simulink model "switch_basic"  (Simulink 6.6)
settings: Solver=FixedStepDiscrete  StartTime=0.0  StopTime=10.0  FixedStep=1  RelTol=1e-3
settings Model: Creator=ksmyth  LastModifiedBy=hnine

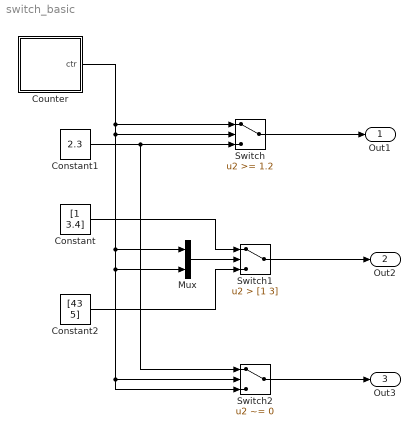
== system switch_basic ==
  Constant : Constant  Value=[1 3.4]
  Constant1 : Constant  Value=2.3
  Constant2 : Constant  Value=[43 5]
  Counter : Stateflow chart
  Mux : Mux  Inputs=2
  Switch : Switch  Threshold=1.2
  Switch1 : Switch  Criteria=u2 > Threshold  Threshold=[1 3]
  Switch2 : Switch  Criteria=u2 ~= 0
  Out1 : Outport
  Out2 : Outport  Port=2
  Out3 : Outport  Port=3
  wires:
  Constant1/1 -> Switch/3, Switch2/1
  Constant/1 -> Switch1/1
  Constant2/1 -> Switch1/3
  Switch/1 -> Out1/1
  Switch1/1 -> Out2/1
  Switch2/1 -> Out3/1
  Counter/1(ctr) -> Switch/2, Mux/1, Switch2/3, Switch2/2, Mux/2, Switch/1
  Mux/1 -> Switch1/2

== stateflow chart Counter ==
  settings: executeAtInitialization=1
  state s1
  (default) -> s1
  s1 -> s1 [order 1] : [ctr < 3] / ctr = ctr+1;
  s1 -> s1 [order 2] : [ctr >= 3] / ctr = 0;
  data: ctr output double =0
